simulink model "TaperedTLMFIRExample"  (R2017b)
settings: Solver=ode23t  StartTime=0.0  StopTime=2  RelTol=1e-6  EnableMultiTasking=on
libraries: usask_tlm_lib x1
settings Model: Creator=Jeremy  LastModifiedBy=tkw954
settings DataIOCC: SaveFormat=Array
settings OptimizationCC: LifeSpan=inf
settings DebuggingCC: SFUnexpectedBacktrackingDiag=warning  SFNoUnconditionalDefaultTransitionDiag=warning  SFExecutionAtInitializationDiag=none
settings HardwareCC: ProdBitPerPointer=32  ProdBitPerSizeT=32  ProdBitPerPtrDiffT=32  ProdLargestAtomicFloat=None  ProdIntDivRoundTo=Undefined  ProdEndianess=Unspecified  ProdWordSize=32  ProdHWDeviceType=32-bit Generic
settings ModelReferenceCC: PropagateSignalLabelsOutOfModel=off
settings CodeAppCC: StateflowObjectComments=on
settings GRTTargetCC: TargetLangStandard=C89/C90 (ANSI)  GeneratePreprocessorConditionals=Disable all
settings ConfigComp: CovMetricSettings=dw  CovHtmlReporting=on  CovSaveCumulativeToWorkspaceVar=on  CovSaveSingleToWorkspaceVar=on  CovExternalEMLEnable=off

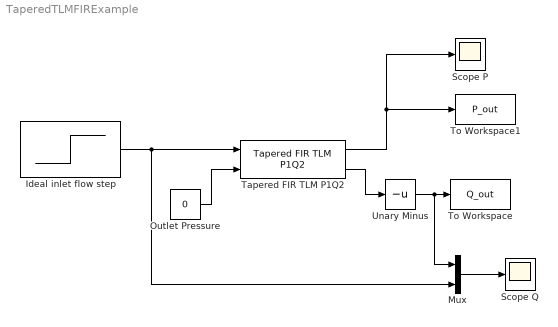
== system TaperedTLMFIRExample ==
  Ideal inlet flow step : Step  After=2.5e-4  SampleTime=0
  Mux : Mux  Inputs=2
  Outlet Pressure : Constant  Value=0
  Scope P : Scope
  Scope Q : Scope
  Tapered FIR TLM P1Q2 : usask_tlm_lib/Tapered FIR TLM P1Q2  D_1=40e-3  D_2=42e-3  L=10  K=1.5e9  nu=100e-6  rho=890
      settings: SourceProductName=USask Transmission Line Model Library
  To Workspace : ToWorkspace  VariableName=Q_out  SampleTime=-1
  To Workspace1 : ToWorkspace  VariableName=P_out  SampleTime=-1
  Unary Minus : UnaryMinus
  wires:
  Ideal inlet flow step/1 -> Tapered FIR TLM P1Q2/1, Mux/2
  Outlet Pressure/1 -> Tapered FIR TLM P1Q2/2
  Tapered FIR TLM P1Q2/1 -> To Workspace1/1, Scope P/1
  Unary Minus/1 -> Mux/1, To Workspace/1
  Mux/1 -> Scope Q/1
  Tapered FIR TLM P1Q2/2 -> Unary Minus/1
